simulink model "fft32kpt_ssr32_float"  (R2024a)
settings: Solver=VariableStepAuto  StartTime=0.0  StopTime=sample_period*N*6  RelTol=1e-3
PreLoadFcn:
  | clk_freq = 570e6;
  | SSR=32; % transpose block SSR settings...
  | sample_period = 1/(SSR*clk_freq);
  | N=32768; % fft point size
  | binw=(1/sample_period) / (2*N); % bin width
  | bin_freq = 2*pi*3*binw+pi*binw; % sin, cos freq centered in channel
  | 
  | % for transpose block
  | DATA_WIDTH=32;
  | M=32;
  | N1=N/M;
  | MEM_STYLE=4; % MEM OPTIONS: 4 - ULTRA, 0 - AUTO, 1 - BRAM, 5 - MIXED
InitFcn:
  | clk_freq = 570e6;
  | SSR=32; % transpose block SSR settings...
  | sample_period = 1/(SSR*clk_freq);
  | N=32768; % fft point size
  | binw=(1/sample_period) / (2*N); % bin width
  | bin_freq = 2*pi*3*binw+pi*binw; % sin, cos freq centered in channel
  | 
  | % for transpose block
  | DATA_WIDTH=32;
  | M=32;
  | N1=N/M;
  | MEM_STYLE=4; % MEM OPTIONS: 4 - ULTRA, 0 - AUTO, 1 - BRAM, 5 - MIXED
undefined symbols (not defined in the file or in its folder): None, S, vsva2197, xcvc1902
libraries: hdlBasic x139, aieBasic x95, aieUtilities x32, aieDSP x32, hdlUtilities x32, matrix_library x32, hdlSSR x12, hdlDSPIP x1, simulink x1, dspxfrm3 x1, vmcUtilities x1
(part 1 of 4)
settings Model: Creator=mmi  LastModifiedBy=robg
settings DebuggingCC: UnconnectedInputMsg=warning  UnconnectedOutputMsg=warning  UnconnectedLineMsg=warning
settings ModelReferenceCC: EnableRefExpFcnMdlSchedulingChecks=on
settings RTWCC: GPUComputeCapability=3.5  DLArmComputeVersion=19.05
settings ConfigComp: CovBoundaryAbsTol=1.0e-5

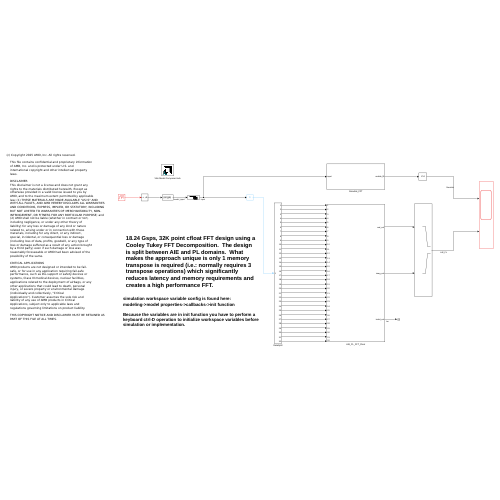
[thumbnail: Simulink's stored preview of the top-level diagram]
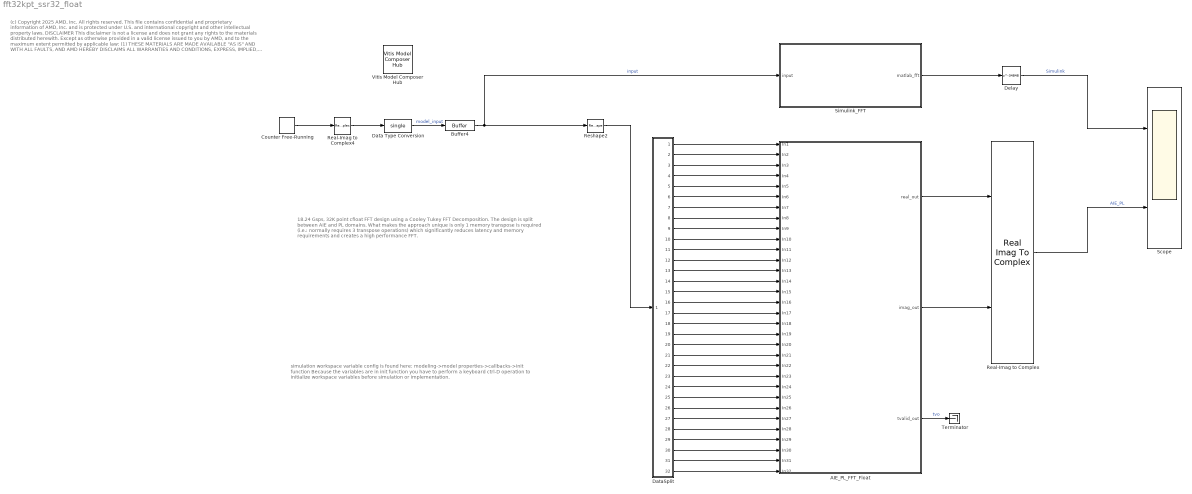
== system fft32kpt_ssr32_float ==
  note: 18.24 Gsps, 32K point cfloat FFT design using a Cooley Tukey FFT Decomposition. The design is split between AIE and PL domains. What makes the approach unique is only 1 memory transpose is required (i.e.: normally requires 3 transpose operations) which significantly reduces latency and memory requirements and creates a high performance FFT.
  note: (c) Copyright 2025 AMD, Inc. All rights reserved.
      |
      | This file contains confidential and proprietary information
      | of AMD, Inc. and is protected under U.S. and
      | international copyright and other intellectual property
      | laws.
      |
      | DISCLAIMER
      | This disclaimer is not a license and does not grant any
      | rights to the materials distributed herewith. Except as
      | otherwise provided in a valid license issued to you by
      | AMD, and to the maximum extent permitted by applicable
      | law: (1) THESE MATERIALS ARE MADE AVAILABLE "AS IS" AND
      | WITH ALL FAULTS, AND AMD HEREBY DISCLAIMS ALL WARRANTIES
      | AND CONDITIONS, EXPRESS, IMPLIED, OR STATUTORY, INCLUDING
      | BUT NOT LIMITED TO WARRANTIES OF MERCHANTABILITY, NON-
      | INFRINGEMENT, OR FITNESS FOR ANY PARTICULAR PURPOSE; and
      | (2) AMD shall not be liable (whether in contract or tort,
      | including negligence, or under any other theory of
      | liability) for any loss or damage of any kind or nature
      | related to, arising under or in connection with these
      | materials, including for any direct, or any indirect,
      | special, incidental, or consequential loss or damage
      | (including loss of data, profits, goodwill, or any type of
      | loss or damage suffered as a result of any action brought
      | by a third party) even if such damage or loss was
      | reasonably foreseeable or AMD had been advised of the
      | possibility of the same.
      |
      | CRITICAL APPLICATIONS
      | AMD products are not designed or intended to be fail-
      | safe, or for use in any application requiring fail-safe
      | performance, such as life-support or safety devices or
      | systems, Class III medical devices, nuclear facilities,
      | applications related to the deployment of airbags, or any
      | other applications that could lead to death, personal
      | injury, or severe property or environmental damage
      | (individually and collectively, "Critical
      | Applications"). Customer assumes the sole risk and
      | liability of any use of AMD products in Critical
      | Applications, subject only to applicable laws and
      | regulations governing limitations on product liability.
      |
      | THIS COPYRIGHT NOTICE AND DISCLAIMER MUST BE RETAINED AS
      | PART OF THIS FILE AT ALL TIMES.
  note: simulation workspace variable config is found here:
      | modeling->model properties->callbacks->init function
      |
      | Because the variables are in init function you have to perform a keyboard ctrl-D operation to initialize workspace variables before simulation or implementation.
  AIE_PL_FFT_Float : Subsystem
  Buffer4 : Buffer  N=N  OutputFrames=off
  Counter Free-Running : simulink/Sources/Counter Free-Running  NumBits=log2(N)  tsamp=sample_period
  Data Type Conversion : DataTypeConversion  OutDataTypeStr=single  SaturateOnIntegerOverflow=off  RndMeth=Floor
  DataSplit : Subsystem
  Delay : Delay  DelayLength=34848
  Real-Imag to Complex : RealImagToComplex
  Real-Imag to Complex4 : RealImagToComplex  Input=Real
  Reshape2 : Reshape  OutputDimensionality=Customize  OutputDimensions=[32,N/32]
  Scope : Scope  NumInputPorts=2
  Simulink_FFT : Subsystem
  Terminator : Terminator
  Vitis Model Composer Hub : vmcUtilities/Vitis Model Composer Hub  Tag=genX  CodeGeneration=off  SubsystemName=FFTs_complexRot  BlockHierPath=fft32kpt_ssr32_float/AIE_PL_FFT_Float/FFTs_complexRot  SubsystemType=AIENode  StartColumn=1  NumberOfColumns=1  TargetDirectory=./code  exportDesign=off  analyzeDesign=on  validateDesignOnHw=off  ExportType=AI Engines  IpVendor=xilinx.com  IpLibrary=hls  IpVersion=1.0  IpHWLanguage=Verilog  AieCompilerOptions={}  AieSimulatorOptions={}  CreateTestbench=on  TestbenchStackSize=10  RunRtlSim=off  RunCSim=off  RunAieSim=on  AieSimTimeout=75000  RunAieSimProfiling=off  LaunchVitisAnalyzer=on  PlotOutput=on  RunX86Sim=off  X86SimTimeout=10  GenHwImage=off  GenLibadfXo=off  GenHwValidationCode=off  PlatformType=Not Specified  HwSystemType=Baremetal  HwValidationTarget=hw  ProjDevice=Versal VCK190 Evaluation Platform with New SD Level Shifter (xcvc1902-vsva2197-2MP-e-S)  ProjDevicePart=xcvc1902-vsva2197-2MP-e-S  AIEType=AIE  SamplePeriod=-1  ClockFrequency=200  DataPathParallelism=1  xilinxfamily=versalaicore  part=xcvc1902  speed=-2MP-e-S  package=vsva2197  directory=./netlist/ip/HDL_32ptFFT_transpose/src  testbench=off  incr_netlist=off  synthesis_tool=Vivado  clock_wrapper=Clock Enables  dbl_ovrd=According to Block Masks  dcm_input_clock_period=10  sysclk_period=1e9/clk_freq  simulink_period=1/clk_freq  eval_field=0  IPInfoJsonString="{\"DUTSubsystemName\":\"FFTs_complexRot\",\"AIESubsystem\":{\"SubsystemName\":\"FFTs_complexRot\",\"TargetDirectory\":\"./code\",\"AIEArrayConfig\":\"Use entire AIE array\",\"StartColumn\":\"0\",\"NumberOfColumns\":\"1\"},\"SubsystemTag\":\"AIENode\"}"  LogFileName=/group/xcoswmktg2/robg/git/vmc_examples/github/Examples/AIENGINE_plus_PL/AIE_HDL/VersalFFT/code/model_composer.log  NThreads=4  IPConfigFile=/tmp/vmctmp-15755458006881932690/fft32kpt_ssr32_float_ipconfig.json
  wires:
  Buffer4/1 -> Simulink_FFT/1(input), Reshape2/1  "input"
  Counter Free-Running/1 -> Real-Imag to Complex4/1
  DataSplit/1(Out1) -> AIE_PL_FFT_Float/1(In1)
  DataSplit/2(Out2) -> AIE_PL_FFT_Float/2(In2)
  DataSplit/3(Out3) -> AIE_PL_FFT_Float/3(In3)
  DataSplit/4(Out4) -> AIE_PL_FFT_Float/4(In4)
  DataSplit/5(Out5) -> AIE_PL_FFT_Float/5(In5)
  DataSplit/6(Out6) -> AIE_PL_FFT_Float/6(In6)
  DataSplit/7(Out7) -> AIE_PL_FFT_Float/7(In7)
  DataSplit/8(Out8) -> AIE_PL_FFT_Float/8(In8)
  DataSplit/9(Out9) -> AIE_PL_FFT_Float/9(In9)
  DataSplit/10(Out10) -> AIE_PL_FFT_Float/10(In10)
  DataSplit/11(Out11) -> AIE_PL_FFT_Float/11(In11)
  DataSplit/12(Out12) -> AIE_PL_FFT_Float/12(In12)
  DataSplit/13(Out13) -> AIE_PL_FFT_Float/13(In13)
  DataSplit/14(Out14) -> AIE_PL_FFT_Float/14(In14)
  DataSplit/15(Out15) -> AIE_PL_FFT_Float/15(In15)
  DataSplit/16(Out16) -> AIE_PL_FFT_Float/16(In16)
  DataSplit/17(Out17) -> AIE_PL_FFT_Float/17(In17)
  DataSplit/18(Out18) -> AIE_PL_FFT_Float/18(In18)
  DataSplit/19(Out19) -> AIE_PL_FFT_Float/19(In19)
  DataSplit/20(Out20) -> AIE_PL_FFT_Float/20(In20)
  DataSplit/21(Out21) -> AIE_PL_FFT_Float/21(In21)
  DataSplit/22(Out22) -> AIE_PL_FFT_Float/22(In22)
  DataSplit/23(Out23) -> AIE_PL_FFT_Float/23(In23)
  DataSplit/24(Out24) -> AIE_PL_FFT_Float/24(In24)
  DataSplit/25(Out25) -> AIE_PL_FFT_Float/25(In25)
  DataSplit/26(Out26) -> AIE_PL_FFT_Float/26(In26)
  DataSplit/27(Out27) -> AIE_PL_FFT_Float/27(In27)
  DataSplit/28(Out28) -> AIE_PL_FFT_Float/28(In28)
  DataSplit/29(Out29) -> AIE_PL_FFT_Float/29(In29)
  DataSplit/30(Out30) -> AIE_PL_FFT_Float/30(In30)
  DataSplit/31(Out31) -> AIE_PL_FFT_Float/31(In31)
  DataSplit/32(Out32) -> AIE_PL_FFT_Float/32(In32)
  Real-Imag to Complex4/1 -> Data Type Conversion/1
  AIE_PL_FFT_Float/1(real_out) -> Real-Imag to Complex/1
  AIE_PL_FFT_Float/2(imag_out) -> Real-Imag to Complex/2
  Data Type Conversion/1 -> Buffer4/1  "model_input"
  Reshape2/1 -> DataSplit/1(In1)
  Delay/1 -> Scope/1  "Simulink"
  Real-Imag to Complex/1 -> Scope/2  "AIE_PL"
  Simulink_FFT/1(matlab_fft) -> Delay/1
  AIE_PL_FFT_Float/3(tvalid_out) -> Terminator/1  "tvo"

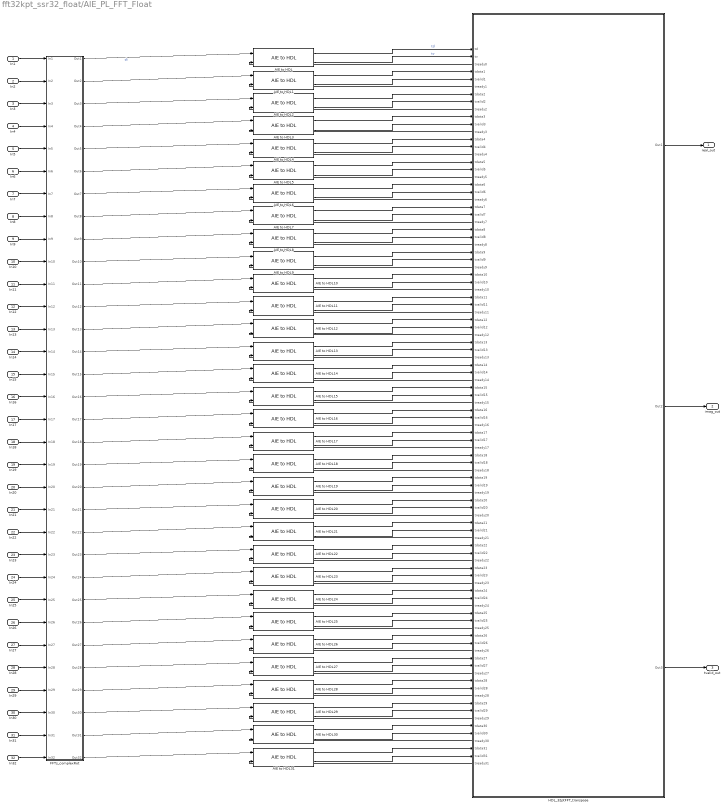
== system fft32kpt_ssr32_float/AIE_PL_FFT_Float ==
  In1 : Inport
  In2 : Inport  Port=2
  In3 : Inport  Port=3
  In4 : Inport  Port=4
  In5 : Inport  Port=5
  In6 : Inport  Port=6
  In7 : Inport  Port=7
  In8 : Inport  Port=8
  In9 : Inport  Port=9
  In10 : Inport  Port=10
  In11 : Inport  Port=11
  In12 : Inport  Port=12
  In13 : Inport  Port=13
  In14 : Inport  Port=14
  In15 : Inport  Port=15
  In16 : Inport  Port=16
  In17 : Inport  Port=17
  In18 : Inport  Port=18
  In19 : Inport  Port=19
  In20 : Inport  Port=20
  In21 : Inport  Port=21
  In22 : Inport  Port=22
  In23 : Inport  Port=23
  In24 : Inport  Port=24
  In25 : Inport  Port=25
  In26 : Inport  Port=26
  In27 : Inport  Port=27
  In28 : Inport  Port=28
  In29 : Inport  Port=29
  In30 : Inport  Port=30
  In31 : Inport  Port=31
  In32 : Inport  Port=32
  AIE to HDL{,1..31} (32 alike) : aieUtilities/AIE to HDL  OutDataType=uint64  OutSampleTime=Inherit: Same as tready
  FFTs_complexRot : Subsystem
  HDL_32ptFFT_transpose : Subsystem
      settings: PortSchema="{\"entries\":[{\"content\":{\"sides\":[{\"content\":{\"connectorIds\":[\"In1\",\"In2\",\"Out4\",\"In3\",\"In4\",\"Out5\",\"In5\",\"In6\",\"Out6\",\"In7\",\"In8\",\"Out7\",\"In9\",\"In10\",\"Out8\",\"In11\",\"In12\",\"Out9\",\"In13\",\"In14\",\"Out10\",\"In15\",\"In16\",\"Out11\",\"In17\",\"In18\",\"Out12\",\"In19\",\"In20\",\"Out13\",\"In21\",\"In22\",\"Out14\",\"In23\",\"In24\",\"Out15\",\"In25\",\"In26\",\"Out16\",\"In27\",\"In28\",\"Out17\",\"In29\",\"In30\",\"Out18\",\"In31\",\"In32\",\"Out19\",\"In33\",\"In34\",\"Out20\",\"In35\",\"In36\",\"Out21\",\"In37\",\"In38\",\"Out22\",\"In39\",\"In40\",\"Out23\",\"In41\",\"In42\",\"Out24\",\"In43\",\"In44\",\"Out25\",\"In45\",\"In46\",\"Out26\",\"In47\",\"In48\",\"Out27\",\"In49\",\"In50\",\"Out28\",\"In51\",\"In52\",\"Out29\",\"In53\",\"In54\",\"Out30\",\"In55\",\"In56\",\"Out31\",\"In57\",\"In58\",\"Out32\",\"In59\",\"In60\",\"Out33\",\"In61\",\"In62\",\"Out34\",\"In63\",\"In64\",\"Out35\"]},\"type\":\"ConnectorPlacement.EquallySpacedRectSide\",\"uuid\":\"3a67bb84-7466-4c33-a7ce-2d251f0b854b\"},{\"content\":{\"connectorIds\":[\"Out1\",\"Out2\",\"Out3\"],\"side\":\"RIGHT\"},\"type\":\"ConnectorPlacement.EquallySpacedRectSide\",\"uuid\":\"c6d3c8b5-bf8d-4a61-84a6-8f283f97da6c\"},{\"content\":{\"side\":\"TOP\"},\"type\":\"ConnectorPlacement.EquallySpacedRectSide\",\"uuid\":\"81fe714e-4dff-42d4-a162-7e084749adf3\"}]},\"type\":\"ConnectorPlacement.EquallySpacedConnector\",\"uuid\":\"fbc5b95b-ed06-45dd-b395-c44856a8f140\"}],\"packageUris\":[\"http://schema.mathworks.com/mf0/Connector/R2020b\"],\"version\":\"1.0\"}"
  real_out : Outport
  imag_out : Outport  Port=2
  tvalid_out : Outport  Port=3
  wires:
  FFTs_complexRot/1(Out1) -> AIE to HDL/1  "di"
  FFTs_complexRot/26(Out26) -> AIE to HDL25/1
  FFTs_complexRot/21(Out21) -> AIE to HDL20/1
  FFTs_complexRot/16(Out16) -> AIE to HDL15/1
  FFTs_complexRot/5(Out5) -> AIE to HDL4/1
  FFTs_complexRot/13(Out13) -> AIE to HDL12/1
  FFTs_complexRot/32(Out32) -> AIE to HDL31/1
  FFTs_complexRot/20(Out20) -> AIE to HDL19/1
  FFTs_complexRot/3(Out3) -> AIE to HDL2/1
  In2/1 -> FFTs_complexRot/2(In2)
  FFTs_complexRot/4(Out4) -> AIE to HDL3/1
  In16/1 -> FFTs_complexRot/16(In16)
  In10/1 -> FFTs_complexRot/10(In10)
  In7/1 -> FFTs_complexRot/7(In7)
  In4/1 -> FFTs_complexRot/4(In4)
  FFTs_complexRot/11(Out11) -> AIE to HDL10/1
  In28/1 -> FFTs_complexRot/28(In28)
  FFTs_complexRot/28(Out28) -> AIE to HDL27/1
  In12/1 -> FFTs_complexRot/12(In12)
  FFTs_complexRot/31(Out31) -> AIE to HDL30/1
  FFTs_complexRot/6(Out6) -> AIE to HDL5/1
  In21/1 -> FFTs_complexRot/21(In21)
  FFTs_complexRot/25(Out25) -> AIE to HDL24/1
  In26/1 -> FFTs_complexRot/26(In26)
  In5/1 -> FFTs_complexRot/5(In5)
  In3/1 -> FFTs_complexRot/3(In3)
  In24/1 -> FFTs_complexRot/24(In24)
  FFTs_complexRot/29(Out29) -> AIE to HDL28/1
  In8/1 -> FFTs_complexRot/8(In8)
  FFTs_complexRot/24(Out24) -> AIE to HDL23/1
  In29/1 -> FFTs_complexRot/29(In29)
  In20/1 -> FFTs_complexRot/20(In20)
  FFTs_complexRot/9(Out9) -> AIE to HDL8/1
  In23/1 -> FFTs_complexRot/23(In23)
  In31/1 -> FFTs_complexRot/31(In31)
  In11/1 -> FFTs_complexRot/11(In11)
  FFTs_complexRot/15(Out15) -> AIE to HDL14/1
  In13/1 -> FFTs_complexRot/13(In13)
  FFTs_complexRot/14(Out14) -> AIE to HDL13/1
  In19/1 -> FFTs_complexRot/19(In19)
  In32/1 -> FFTs_complexRot/32(In32)
  In17/1 -> FFTs_complexRot/17(In17)
  In22/1 -> FFTs_complexRot/22(In22)
  FFTs_complexRot/17(Out17) -> AIE to HDL16/1
  In30/1 -> FFTs_complexRot/30(In30)
  In27/1 -> FFTs_complexRot/27(In27)
  In18/1 -> FFTs_complexRot/18(In18)
  FFTs_complexRot/19(Out19) -> AIE to HDL18/1
  In14/1 -> FFTs_complexRot/14(In14)
  In9/1 -> FFTs_complexRot/9(In9)
  FFTs_complexRot/8(Out8) -> AIE to HDL7/1
  FFTs_complexRot/2(Out2) -> AIE to HDL1/1
  FFTs_complexRot/10(Out10) -> AIE to HDL9/1
  FFTs_complexRot/22(Out22) -> AIE to HDL21/1
  In15/1 -> FFTs_complexRot/15(In15)
  FFTs_complexRot/27(Out27) -> AIE to HDL26/1
  FFTs_complexRot/12(Out12) -> AIE to HDL11/1
  FFTs_complexRot/23(Out23) -> AIE to HDL22/1
  FFTs_complexRot/30(Out30) -> AIE to HDL29/1
  In6/1 -> FFTs_complexRot/6(In6)
  In25/1 -> FFTs_complexRot/25(In25)
  In1/1 -> FFTs_complexRot/1(In1)
  FFTs_complexRot/7(Out7) -> AIE to HDL6/1
  FFTs_complexRot/18(Out18) -> AIE to HDL17/1
  AIE to HDL/1 -> HDL_32ptFFT_transpose/1(td)  "td"
  AIE to HDL/2 -> HDL_32ptFFT_transpose/2(tv)  "tv"
  AIE to HDL1/1 -> HDL_32ptFFT_transpose/3(tdata1)
  AIE to HDL1/2 -> HDL_32ptFFT_transpose/4(tvalid1)
  AIE to HDL2/1 -> HDL_32ptFFT_transpose/5(tdata2)
  AIE to HDL2/2 -> HDL_32ptFFT_transpose/6(tvalid2)
  AIE to HDL3/1 -> HDL_32ptFFT_transpose/7(tdata3)
  AIE to HDL3/2 -> HDL_32ptFFT_transpose/8(tvalid3)
  AIE to HDL4/1 -> HDL_32ptFFT_transpose/9(tdata4)
  AIE to HDL4/2 -> HDL_32ptFFT_transpose/10(tvalid4)
  AIE to HDL5/1 -> HDL_32ptFFT_transpose/11(tdata5)
  AIE to HDL5/2 -> HDL_32ptFFT_transpose/12(tvalid5)
  AIE to HDL6/1 -> HDL_32ptFFT_transpose/13(tdata6)
  AIE to HDL6/2 -> HDL_32ptFFT_transpose/14(tvalid6)
  AIE to HDL7/1 -> HDL_32ptFFT_transpose/15(tdata7)
  AIE to HDL7/2 -> HDL_32ptFFT_transpose/16(tvalid7)
  AIE to HDL8/1 -> HDL_32ptFFT_transpose/17(tdata8)
  AIE to HDL8/2 -> HDL_32ptFFT_transpose/18(tvalid8)
  AIE to HDL9/1 -> HDL_32ptFFT_transpose/19(tdata9)
  AIE to HDL9/2 -> HDL_32ptFFT_transpose/20(tvalid9)
  AIE to HDL10/1 -> HDL_32ptFFT_transpose/21(tdata10)
  AIE to HDL10/2 -> HDL_32ptFFT_transpose/22(tvalid10)
  AIE to HDL11/1 -> HDL_32ptFFT_transpose/23(tdata11)
  AIE to HDL11/2 -> HDL_32ptFFT_transpose/24(tvalid11)
  AIE to HDL12/1 -> HDL_32ptFFT_transpose/25(tdata12)
  AIE to HDL12/2 -> HDL_32ptFFT_transpose/26(tvalid12)
  AIE to HDL13/1 -> HDL_32ptFFT_transpose/27(tdata13)
  AIE to HDL13/2 -> HDL_32ptFFT_transpose/28(tvalid13)
  AIE to HDL14/1 -> HDL_32ptFFT_transpose/29(tdata14)
  AIE to HDL14/2 -> HDL_32ptFFT_transpose/30(tvalid14)
  AIE to HDL15/1 -> HDL_32ptFFT_transpose/31(tdata15)
  AIE to HDL15/2 -> HDL_32ptFFT_transpose/32(tvalid15)
  AIE to HDL16/1 -> HDL_32ptFFT_transpose/33(tdata16)
  AIE to HDL16/2 -> HDL_32ptFFT_transpose/34(tvalid16)
  AIE to HDL17/1 -> HDL_32ptFFT_transpose/35(tdata17)
  AIE to HDL17/2 -> HDL_32ptFFT_transpose/36(tvalid17)
  AIE to HDL18/1 -> HDL_32ptFFT_transpose/37(tdata18)
  AIE to HDL18/2 -> HDL_32ptFFT_transpose/38(tvalid18)
  AIE to HDL19/1 -> HDL_32ptFFT_transpose/39(tdata19)
  AIE to HDL19/2 -> HDL_32ptFFT_transpose/40(tvalid19)
  AIE to HDL20/1 -> HDL_32ptFFT_transpose/41(tdata20)
  AIE to HDL20/2 -> HDL_32ptFFT_transpose/42(tvalid20)
  AIE to HDL21/1 -> HDL_32ptFFT_transpose/43(tdata21)
  AIE to HDL21/2 -> HDL_32ptFFT_transpose/44(tvalid21)
  AIE to HDL22/1 -> HDL_32ptFFT_transpose/45(tdata22)
  AIE to HDL22/2 -> HDL_32ptFFT_transpose/46(tvalid22)
  AIE to HDL23/1 -> HDL_32ptFFT_transpose/47(tdata23)
  AIE to HDL23/2 -> HDL_32ptFFT_transpose/48(tvalid23)
  AIE to HDL24/1 -> HDL_32ptFFT_transpose/49(tdata24)
  AIE to HDL24/2 -> HDL_32ptFFT_transpose/50(tvalid24)
  AIE to HDL25/1 -> HDL_32ptFFT_transpose/51(tdata25)
  AIE to HDL25/2 -> HDL_32ptFFT_transpose/52(tvalid25)
  AIE to HDL26/1 -> HDL_32ptFFT_transpose/53(tdata26)
  AIE to HDL26/2 -> HDL_32ptFFT_transpose/54(tvalid26)
  AIE to HDL27/1 -> HDL_32ptFFT_transpose/55(tdata27)
  AIE to HDL27/2 -> HDL_32ptFFT_transpose/56(tvalid27)
  AIE to HDL28/1 -> HDL_32ptFFT_transpose/57(tdata28)
  AIE to HDL28/2 -> HDL_32ptFFT_transpose/58(tvalid28)
  AIE to HDL29/1 -> HDL_32ptFFT_transpose/59(tdata29)
  AIE to HDL29/2 -> HDL_32ptFFT_transpose/60(tvalid29)
  AIE to HDL30/1 -> HDL_32ptFFT_transpose/61(tdata30)
  AIE to HDL30/2 -> HDL_32ptFFT_transpose/62(tvalid30)
  AIE to HDL31/1 -> HDL_32ptFFT_transpose/63(tdata31)
  AIE to HDL31/2 -> HDL_32ptFFT_transpose/64(tvalid31)
  HDL_32ptFFT_transpose/1(Out1) -> real_out/1
  HDL_32ptFFT_transpose/2(Out2) -> imag_out/1
  HDL_32ptFFT_transpose/3(Out3) -> tvalid_out/1
  HDL_32ptFFT_transpose/4(tready0) -> AIE to HDL/2
  HDL_32ptFFT_transpose/5(tready1) -> AIE to HDL1/2
  HDL_32ptFFT_transpose/6(tready2) -> AIE to HDL2/2
  HDL_32ptFFT_transpose/7(tready3) -> AIE to HDL3/2
  HDL_32ptFFT_transpose/8(tready4) -> AIE to HDL4/2
  HDL_32ptFFT_transpose/9(tready5) -> AIE to HDL5/2
  HDL_32ptFFT_transpose/10(tready6) -> AIE to HDL6/2
  HDL_32ptFFT_transpose/11(tready7) -> AIE to HDL7/2
  HDL_32ptFFT_transpose/12(tready8) -> AIE to HDL8/2
  HDL_32ptFFT_transpose/13(tready9) -> AIE to HDL9/2
  HDL_32ptFFT_transpose/14(tready10) -> AIE to HDL10/2
  HDL_32ptFFT_transpose/15(tready11) -> AIE to HDL11/2
  HDL_32ptFFT_transpose/16(tready12) -> AIE to HDL12/2
  HDL_32ptFFT_transpose/17(tready13) -> AIE to HDL13/2
  HDL_32ptFFT_transpose/18(tready14) -> AIE to HDL14/2
  HDL_32ptFFT_transpose/19(tready15) -> AIE to HDL15/2
  HDL_32ptFFT_transpose/20(tready16) -> AIE to HDL16/2
  HDL_32ptFFT_transpose/21(tready17) -> AIE to HDL17/2
  HDL_32ptFFT_transpose/22(tready18) -> AIE to HDL18/2
  HDL_32ptFFT_transpose/23(tready19) -> AIE to HDL19/2
  HDL_32ptFFT_transpose/24(tready20) -> AIE to HDL20/2
  HDL_32ptFFT_transpose/25(tready21) -> AIE to HDL21/2
  HDL_32ptFFT_transpose/26(tready22) -> AIE to HDL22/2
  HDL_32ptFFT_transpose/27(tready23) -> AIE to HDL23/2
  HDL_32ptFFT_transpose/28(tready24) -> AIE to HDL24/2
  HDL_32ptFFT_transpose/29(tready25) -> AIE to HDL25/2
  HDL_32ptFFT_transpose/30(tready26) -> AIE to HDL26/2
  HDL_32ptFFT_transpose/31(tready27) -> AIE to HDL27/2
  HDL_32ptFFT_transpose/32(tready28) -> AIE to HDL28/2
  HDL_32ptFFT_transpose/33(tready29) -> AIE to HDL29/2
  HDL_32ptFFT_transpose/34(tready30) -> AIE to HDL30/2
  HDL_32ptFFT_transpose/35(tready31) -> AIE to HDL31/2

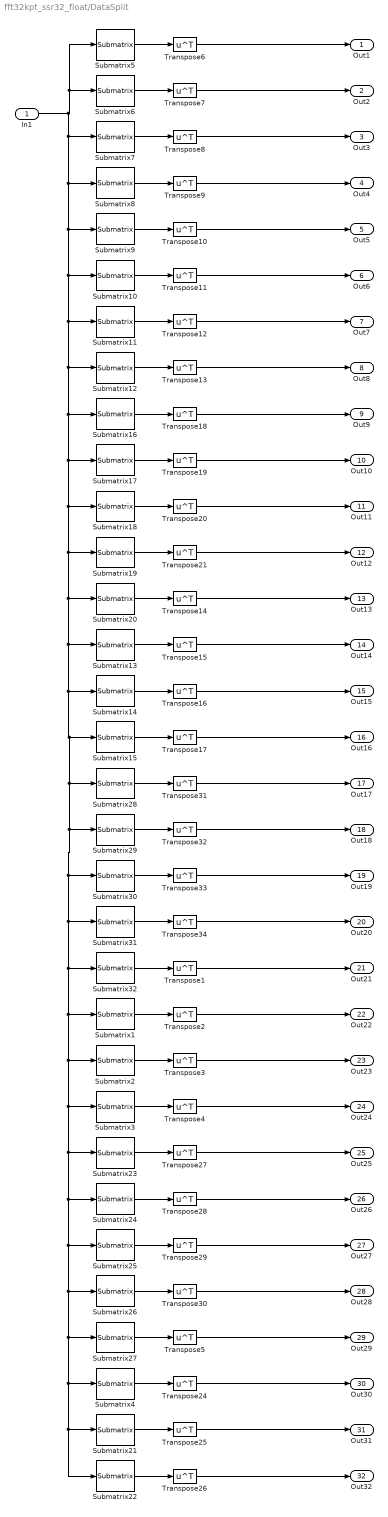
== system fft32kpt_ssr32_float/DataSplit ==
  In1 : Inport
  Submatrix1 : matrix_library/Submatrix  RowSpan=One row  RowStartMode=Index  RowStartIndex=22  RowEndMode=Last  RowEndIndex=1  ColSpan=Range of columns  ColStartMode=First  ColStartIndex=1  ColEndMode=Last  ColEndIndex=1
  Submatrix10 : matrix_library/Submatrix  RowSpan=One row  RowStartMode=Index  RowStartIndex=6  RowEndMode=Last  RowEndIndex=1  ColSpan=Range of columns  ColStartMode=First  ColStartIndex=1  ColEndMode=Last  ColEndIndex=1
  Submatrix11 : matrix_library/Submatrix  RowSpan=One row  RowStartMode=Index  RowStartIndex=7  RowEndMode=Last  RowEndIndex=1  ColSpan=Range of columns  ColStartMode=First  ColStartIndex=1  ColEndMode=Last  ColEndIndex=1
  Submatrix12 : matrix_library/Submatrix  RowSpan=One row  RowStartMode=Index  RowStartIndex=8  RowEndMode=Last  RowEndIndex=1  ColSpan=Range of columns  ColStartMode=First  ColStartIndex=1  ColEndMode=Last  ColEndIndex=1
  Submatrix13 : matrix_library/Submatrix  RowSpan=One row  RowStartMode=Index  RowStartIndex=14  RowEndMode=Last  RowEndIndex=1  ColSpan=Range of columns  ColStartMode=First  ColStartIndex=1  ColEndMode=Last  ColEndIndex=1
  Submatrix14 : matrix_library/Submatrix  RowSpan=One row  RowStartMode=Index  RowStartIndex=15  RowEndMode=Last  RowEndIndex=1  ColSpan=Range of columns  ColStartMode=First  ColStartIndex=1  ColEndMode=Last  ColEndIndex=1
  Submatrix15 : matrix_library/Submatrix  RowSpan=One row  RowStartMode=Index  RowStartIndex=16  RowEndMode=Last  RowEndIndex=1  ColSpan=Range of columns  ColStartMode=First  ColStartIndex=1  ColEndMode=Last  ColEndIndex=1
  Submatrix16 : matrix_library/Submatrix  RowSpan=One row  RowStartMode=Index  RowStartIndex=9  RowEndMode=Last  RowEndIndex=1  ColSpan=Range of columns  ColStartMode=First  ColStartIndex=1  ColEndMode=Last  ColEndIndex=1
  Submatrix17 : matrix_library/Submatrix  RowSpan=One row  RowStartMode=Index  RowStartIndex=10  RowEndMode=Last  RowEndIndex=1  ColSpan=Range of columns  ColStartMode=First  ColStartIndex=1  ColEndMode=Last  ColEndIndex=1
  Submatrix18 : matrix_library/Submatrix  RowSpan=One row  RowStartMode=Index  RowStartIndex=11  RowEndMode=Last  RowEndIndex=1  ColSpan=Range of columns  ColStartMode=First  ColStartIndex=1  ColEndMode=Last  ColEndIndex=1
  Submatrix19 : matrix_library/Submatrix  RowSpan=One row  RowStartMode=Index  RowStartIndex=12  RowEndMode=Last  RowEndIndex=1  ColSpan=Range of columns  ColStartMode=First  ColStartIndex=1  ColEndMode=Last  ColEndIndex=1
  Submatrix2 : matrix_library/Submatrix  RowSpan=One row  RowStartMode=Index  RowStartIndex=23  RowEndMode=Last  RowEndIndex=1  ColSpan=Range of columns  ColStartMode=First  ColStartIndex=1  ColEndMode=Last  ColEndIndex=1
  Submatrix20 : matrix_library/Submatrix  RowSpan=One row  RowStartMode=Index  RowStartIndex=13  RowEndMode=Last  RowEndIndex=1  ColSpan=Range of columns  ColStartMode=First  ColStartIndex=1  ColEndMode=Last  ColEndIndex=1
  Submatrix21 : matrix_library/Submatrix  RowSpan=One row  RowStartMode=Index  RowStartIndex=31  RowEndMode=Last  RowEndIndex=1  ColSpan=Range of columns  ColStartMode=First  ColStartIndex=1  ColEndMode=Last  ColEndIndex=1
  Submatrix22 : matrix_library/Submatrix  RowSpan=One row  RowStartMode=Index  RowStartIndex=32  RowEndMode=Last  RowEndIndex=1  ColSpan=Range of columns  ColStartMode=First  ColStartIndex=1  ColEndMode=Last  ColEndIndex=1
  Submatrix23 : matrix_library/Submatrix  RowSpan=One row  RowStartMode=Index  RowStartIndex=25  RowEndMode=Last  RowEndIndex=1  ColSpan=Range of columns  ColStartMode=First  ColStartIndex=1  ColEndMode=Last  ColEndIndex=1
  Submatrix24 : matrix_library/Submatrix  RowSpan=One row  RowStartMode=Index  RowStartIndex=26  RowEndMode=Last  RowEndIndex=1  ColSpan=Range of columns  ColStartMode=First  ColStartIndex=1  ColEndMode=Last  ColEndIndex=1
  Submatrix25 : matrix_library/Submatrix  RowSpan=One row  RowStartMode=Index  RowStartIndex=27  RowEndMode=Last  RowEndIndex=1  ColSpan=Range of columns  ColStartMode=First  ColStartIndex=1  ColEndMode=Last  ColEndIndex=1
  Submatrix26 : matrix_library/Submatrix  RowSpan=One row  RowStartMode=Index  RowStartIndex=28  RowEndMode=Last  RowEndIndex=1  ColSpan=Range of columns  ColStartMode=First  ColStartIndex=1  ColEndMode=Last  ColEndIndex=1
  Submatrix27 : matrix_library/Submatrix  RowSpan=One row  RowStartMode=Index  RowStartIndex=29  RowEndMode=Last  RowEndIndex=1  ColSpan=Range of columns  ColStartMode=First  ColStartIndex=1  ColEndMode=Last  ColEndIndex=1
  Submatrix28 : matrix_library/Submatrix  RowSpan=One row  RowStartMode=Index  RowStartIndex=17  RowEndMode=Last  RowEndIndex=1  ColSpan=Range of columns  ColStartMode=First  ColStartIndex=1  ColEndMode=Last  ColEndIndex=1
  Submatrix29 : matrix_library/Submatrix  RowSpan=One row  RowStartMode=Index  RowStartIndex=18  RowEndMode=Last  RowEndIndex=1  ColSpan=Range of columns  ColStartMode=First  ColStartIndex=1  ColEndMode=Last  ColEndIndex=1
  Submatrix3 : matrix_library/Submatrix  RowSpan=One row  RowStartMode=Index  RowStartIndex=24  RowEndMode=Last  RowEndIndex=1  ColSpan=Range of columns  ColStartMode=First  ColStartIndex=1  ColEndMode=Last  ColEndIndex=1
  Submatrix30 : matrix_library/Submatrix  RowSpan=One row  RowStartMode=Index  RowStartIndex=19  RowEndMode=Last  RowEndIndex=1  ColSpan=Range of columns  ColStartMode=First  ColStartIndex=1  ColEndMode=Last  ColEndIndex=1
  Submatrix31 : matrix_library/Submatrix  RowSpan=One row  RowStartMode=Index  RowStartIndex=20  RowEndMode=Last  RowEndIndex=1  ColSpan=Range of columns  ColStartMode=First  ColStartIndex=1  ColEndMode=Last  ColEndIndex=1
  Submatrix32 : matrix_library/Submatrix  RowSpan=One row  RowStartMode=Index  RowStartIndex=21  RowEndMode=Last  RowEndIndex=1  ColSpan=Range of columns  ColStartMode=First  ColStartIndex=1  ColEndMode=Last  ColEndIndex=1
  Submatrix4 : matrix_library/Submatrix  RowSpan=One row  RowStartMode=Index  RowStartIndex=30  RowEndMode=Last  RowEndIndex=1  ColSpan=Range of columns  ColStartMode=First  ColStartIndex=1  ColEndMode=Last  ColEndIndex=1
  Submatrix5 : matrix_library/Submatrix  RowSpan=One row  RowStartMode=First  RowStartIndex=1  RowEndMode=Last  RowEndIndex=1  ColSpan=Range of columns  ColStartMode=First  ColStartIndex=1  ColEndMode=Last  ColEndIndex=1
  Submatrix6 : matrix_library/Submatrix  RowSpan=One row  RowStartMode=Index  RowStartIndex=2  RowEndMode=Last  RowEndIndex=1  ColSpan=Range of columns  ColStartMode=First  ColStartIndex=1  ColEndMode=Last  ColEndIndex=1
  Submatrix7 : matrix_library/Submatrix  RowSpan=One row  RowStartMode=Index  RowStartIndex=3  RowEndMode=Last  RowEndIndex=1  ColSpan=Range of columns  ColStartMode=First  ColStartIndex=1  ColEndMode=Last  ColEndIndex=1
  Submatrix8 : matrix_library/Submatrix  RowSpan=One row  RowStartMode=Index  RowStartIndex=4  RowEndMode=Last  RowEndIndex=1  ColSpan=Range of columns  ColStartMode=First  ColStartIndex=1  ColEndMode=Last  ColEndIndex=1
  Submatrix9 : matrix_library/Submatrix  RowSpan=One row  RowStartMode=Index  RowStartIndex=5  RowEndMode=Last  RowEndIndex=1  ColSpan=Range of columns  ColStartMode=First  ColStartIndex=1  ColEndMode=Last  ColEndIndex=1
  Transpose{1..21,24..34} (32 alike) : Math  Operator=transpose
  Out1 : Outport
  Out2 : Outport  Port=2
  Out3 : Outport  Port=3
  Out4 : Outport  Port=4
  Out5 : Outport  Port=5
  Out6 : Outport  Port=6
  Out7 : Outport  Port=7
  Out8 : Outport  Port=8
  Out9 : Outport  Port=9
  Out10 : Outport  Port=10
  Out11 : Outport  Port=11
  Out12 : Outport  Port=12
  Out13 : Outport  Port=13
  Out14 : Outport  Port=14
  Out15 : Outport  Port=15
  Out16 : Outport  Port=16
  Out17 : Outport  Port=17
  Out18 : Outport  Port=18
  Out19 : Outport  Port=19
  Out20 : Outport  Port=20
  Out21 : Outport  Port=21
  Out22 : Outport  Port=22
  Out23 : Outport  Port=23
  Out24 : Outport  Port=24
  Out25 : Outport  Port=25
  Out26 : Outport  Port=26
  Out27 : Outport  Port=27
  Out28 : Outport  Port=28
  Out29 : Outport  Port=29
  Out30 : Outport  Port=30
  Out31 : Outport  Port=31
  Out32 : Outport  Port=32
  wires:
  Submatrix18/1 -> Transpose20/1
  Submatrix11/1 -> Transpose12/1
  Submatrix7/1 -> Transpose8/1
  Transpose26/1 -> Out32/1
  Transpose27/1 -> Out25/1
  Submatrix23/1 -> Transpose27/1
  Transpose21/1 -> Out12/1
  Submatrix25/1 -> Transpose29/1
  Transpose30/1 -> Out28/1
  Submatrix3/1 -> Transpose4/1
  Transpose9/1 -> Out4/1
  Transpose18/1 -> Out9/1
  In1/1 -> Submatrix7/1, Submatrix9/1, Submatrix10/1, Submatrix11/1, Submatrix12/1, Submatrix16/1, Submatrix17/1, Submatrix18/1, Submatrix19/1, Submatrix20/1, Submatrix13/1, Submatrix14/1, Submatrix30/1, Submatrix32/1, Submatrix1/1, Submatrix2/1, Submatrix3/1, Submatrix23/1, Submatrix24/1, Submatrix25/1, Submatrix26/1, Submatrix27/1, Submatrix4/1, Submatrix21/1, Submatrix22/1, Submatrix31/1, Submatrix29/1, Submatrix28/1, Submatrix15/1, Submatrix8/1, Submatrix6/1, Submatrix5/1
  Submatrix15/1 -> Transpose17/1
  Transpose15/1 -> Out14/1
  Transpose19/1 -> Out10/1
  Transpose10/1 -> Out5/1
  Submatrix10/1 -> Transpose11/1
  Transpose1/1 -> Out21/1
  Transpose24/1 -> Out30/1
  Submatrix6/1 -> Transpose7/1
  Transpose33/1 -> Out19/1
  Transpose17/1 -> Out16/1
  Transpose5/1 -> Out29/1
  Submatrix13/1 -> Transpose15/1
  Transpose28/1 -> Out26/1
  Transpose16/1 -> Out15/1
  Submatrix5/1 -> Transpose6/1
  Submatrix27/1 -> Transpose5/1
  Transpose12/1 -> Out7/1
  Transpose11/1 -> Out6/1
  Transpose25/1 -> Out31/1
  Submatrix20/1 -> Transpose14/1
  Transpose2/1 -> Out22/1
  Transpose31/1 -> Out17/1
  Transpose6/1 -> Out1/1
  Transpose14/1 -> Out13/1
  Transpose3/1 -> Out23/1
  Submatrix31/1 -> Transpose34/1
  Submatrix30/1 -> Transpose33/1
  Submatrix8/1 -> Transpose9/1
  Transpose34/1 -> Out20/1
  Transpose32/1 -> Out18/1
  Submatrix1/1 -> Transpose2/1
  Submatrix21/1 -> Transpose25/1
  Transpose13/1 -> Out8/1
  Submatrix4/1 -> Transpose24/1
  Submatrix32/1 -> Transpose1/1
  Submatrix24/1 -> Transpose28/1
  Submatrix12/1 -> Transpose13/1
  Submatrix28/1 -> Transpose31/1
  Transpose7/1 -> Out2/1
  Submatrix29/1 -> Transpose32/1
  Transpose8/1 -> Out3/1
  Submatrix14/1 -> Transpose16/1
  Submatrix9/1 -> Transpose10/1
  Submatrix19/1 -> Transpose21/1
  Submatrix22/1 -> Transpose26/1
  Submatrix17/1 -> Transpose19/1
  Transpose29/1 -> Out27/1
  Submatrix26/1 -> Transpose30/1
  Transpose20/1 -> Out11/1
  Submatrix2/1 -> Transpose3/1
  Transpose4/1 -> Out24/1
  Submatrix16/1 -> Transpose18/1

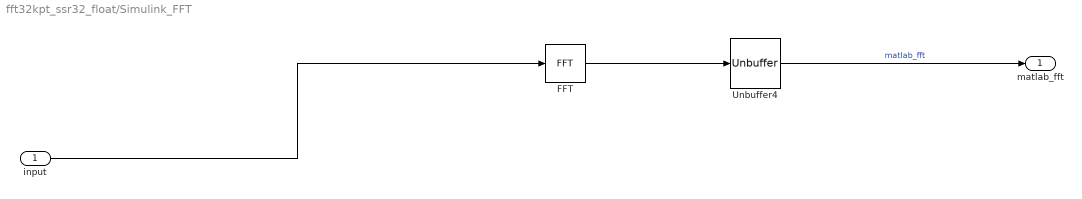
== system fft32kpt_ssr32_float/Simulink_FFT ==
  input : Inport
  FFT : dspxfrm3/FFT  FFTImplementation=Auto  CompMethod=Table lookup  TableOpt=NEW  TableOptActive=Speed  BitRevOrder=off  Normalize=off  InheritFFTLength=on  FFTLength=64  WrapInput=on  roundingMode=Floor  overflowMode=off  firstCoeffDataTypeStr=Inherit: Same word length as input  firstCoeffLastDataTypeStr=Inherit: Same word length as input  outputMin=[]  outputMax=[]
  Unbuffer4 : Unbuffer
  matlab_fft : Outport
  wires:
  FFT/1 -> Unbuffer4/1
  Unbuffer4/1 -> matlab_fft/1  "matlab_fft"
  input/1 -> FFT/1
